simulink model "UnitDelayBio1"  (R2017b)
settings: Solver=FixedStepDiscrete  StartTime=0.0  StopTime=10.0  FixedStep=0.2  RelTol=1e-3  EnableMultiTasking=on
PreLoadFcn:
  | cellInfo =  {
  |   { ...
  |     'acs_command_msg', ...
  |     '', ...
  |     sprintf(''), { ...
  |       {'torque_com_wheel', 3, 'double', -1, 'real', 'Sample'}; ...
  |       {'thruster_on_times', 6, 'double', -1, 'real', 'Sample'}; ...
  |    }
  |   }
  | };
  | Simulink.Bus.cellToObject(cellInfo);
  | 
  | 
  | cellInfo = {
  |     { ...
  |          'command_state_msg' , ...
  |          '', ...
  |          sprintf(''), {  ...
  |                {  'q_com', 4, 'single', -1, 'real', 'Sample' }; ...
  |                {  'sm_spin_axis', 3, 'single', -1, 'real', 'Sample' }; ...
  |                {  'sm_rate_vec', 3, 'single', -1, 'real', 'Sample' }; ...
  |                {  'man_wheel_speed', 3, 'single', -1, 'real', 'Sample' }; ...
  |                {  'man_wheel_torq', 3, 'single', -1, 'real', 'Sample' }; ...
  |                {  'man_gimbal_cmd', 1, 'int16', -1, 'real', 'Sample' }; ...
  |                {  'man_prop_cmd', 8, 'uint16', -1, 'real', 'Sample' }; ...
  |                {  'gyro_LPF_on', 1, 'uint8', -1, 'real', 'Sample' }; ...
  |                {  'st_status', 1, 'uint8', -1, 'real', 'Sample' }; ...
  |                {  'mode', 1, 'uint8', -1, 'real', 'Sample' }; ...
  |                {  'KF_enable', 1, 'uint8', -1, 'real', 'Sample' }; ...
  |                {  'bypass_acs', 3, 'uint8', -1, 'real', 'Sample' }; ...
  |                {  'mm_flag', 1, 'uint8', -1, 'real', 'Sample' }; ...
  |          }
  |     }
  | };
  | Simulink.Bus.cellToObject(cellInfo);
  | 
  | dt = 0.2;
settings Model: Creator=hbourbou  LastModifiedBy=hbourbou
settings DataIOCC: LimitDataPoints=on  SaveFormat=Structure
settings OptimizationCC: LifeSpan=inf
settings DebuggingCC: SFUnexpectedBacktrackingDiag=warning  SFNoUnconditionalDefaultTransitionDiag=warning  SFExecutionAtInitializationDiag=none
settings HardwareCC: ProdBitPerPointer=32  ProdBitPerSizeT=32  ProdBitPerPtrDiffT=32  ProdLargestAtomicFloat=None  ProdIntDivRoundTo=Undefined  ProdEndianess=Unspecified  ProdWordSize=32  ProdHWDeviceType=32-bit Generic
settings ModelReferenceCC: PropagateSignalLabelsOutOfModel=off
settings CodeAppCC: StateflowObjectComments=on
settings GRTTargetCC: TargetLangStandard=C89/C90 (ANSI)  GeneratePreprocessorConditionals=Disable all
settings ConfigComp: CovMetricSettings=dw  CovHtmlReporting=on  CovSaveCumulativeToWorkspaceVar=on  CovSaveSingleToWorkspaceVar=on  CovExternalEMLEnable=off

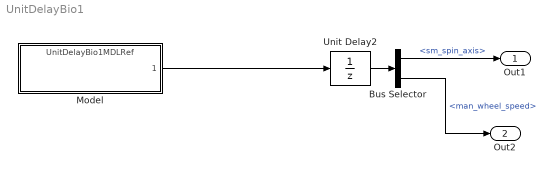
== system UnitDelayBio1 ==
  Bus Selector : BusSelector  OutputSignals=sm_spin_axis,man_wheel_speed
  Model : ModelReference  ModelNameDialog=UnitDelayBio1MDLRef.slx  SimulationMode=Normal  ModelReferenceVersion=1.83
  Unit Delay2 : UnitDelay  SampleTime=-1
  Out1 : Outport
  Out2 : Outport  Port=2
  wires:
  Unit Delay2/1 -> Bus Selector/1
  Bus Selector/1 -> Out1/1  "<sm_spin_axis>"
  Bus Selector/2 -> Out2/1  "<man_wheel_speed>"
  Model/1 -> Unit Delay2/1
